simulink model "ResonantLLCConverter_continuous"  (R2024b)
settings: Solver=FixedStepAuto  StartTime=0.0  StopTime=tfinal  MaxStep=1e-4  RelTol=1e-6  EnableMultiTasking=on
PreLoadFcn:
  | Rs_fet=1e8;  % FET snubber resistance (ohms)
  | Cs_fet=inf;  % FET snubber capacitance (ohms)
  | Vf=0.6;        % Diode forward voltage (V)
libraries: spsDiodeLib x6, spsSeriesRLCBranchLib x3, spsCurrentMeasurementLib x3, spsIGBTDiodeLib x2, spsIdealSwitchLib x2, spsOnDelayLib x2, spsVoltageMeasurementLib x2, spsLinearTransformerLib x1, spsControlledVoltageSourceLib x1, sps_lib x1
settings Model: SimulationMode=accelerator  Creator=The MathWorks, Inc.  LastModifiedBy=XixiLab
settings SolverCC: AlgebraicLoopSolver=TrustRegion  SolverResetMethod=Robust  EnableFixedStepZeroCrossing=on
settings DataIOCC: SaveFormat=Array  SaveState=on  ReturnWorkspaceOutputs=off
settings OptimizationCC: LifeSpan=inf
settings DebuggingCC: ReadBeforeWriteMsg=DisableAll  WriteAfterWriteMsg=DisableAll  WriteAfterReadMsg=DisableAll  MultiTaskDSMMsg=none  UnconnectedInputMsg=warning  UnconnectedOutputMsg=warning  UnconnectedLineMsg=warning  SFUnexpectedBacktrackingDiag=warning  SFNoUnconditionalDefaultTransitionDiag=warning  SFExecutionAtInitializationDiag=none  ArithmeticOperatorsInVariantConditions=warning
settings ModelReferenceCC: UpdateModelReferenceTargets=IfOutOfDate  EnableRefExpFcnMdlSchedulingChecks=on
settings SFSimCC: SFSimEcho=off  SimUseLocalCustomCode=off  CustomCodeUndefinedFunction=UseInterfaceOnly
settings RTWCC: RTWUseLocalCustomCode=off  GPUComputeCapability=3.5
settings CodeAppCC: StateflowObjectComments=on
settings GRTTargetCC: TargetLangStandard=C89/C90 (ANSI)
settings ConfigComp: CovMetricSettings=dw  CovSaveCumulativeToWorkspaceVar=on  CovSaveSingleToWorkspaceVar=on  CovExternalEMLEnable=off
settings SimscapeCC: SimscapeNormalizeSystem=off  SimscapeNominalValues={1, 'bar'; 1, 'cm^3/s'; 1, 'bar*kg/s'; 1, 'kJ/kg'; 1, 'kW'; }

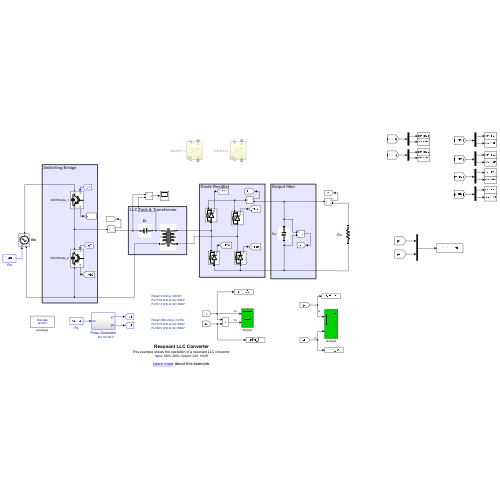
[thumbnail: Simulink's stored preview of the top-level diagram]
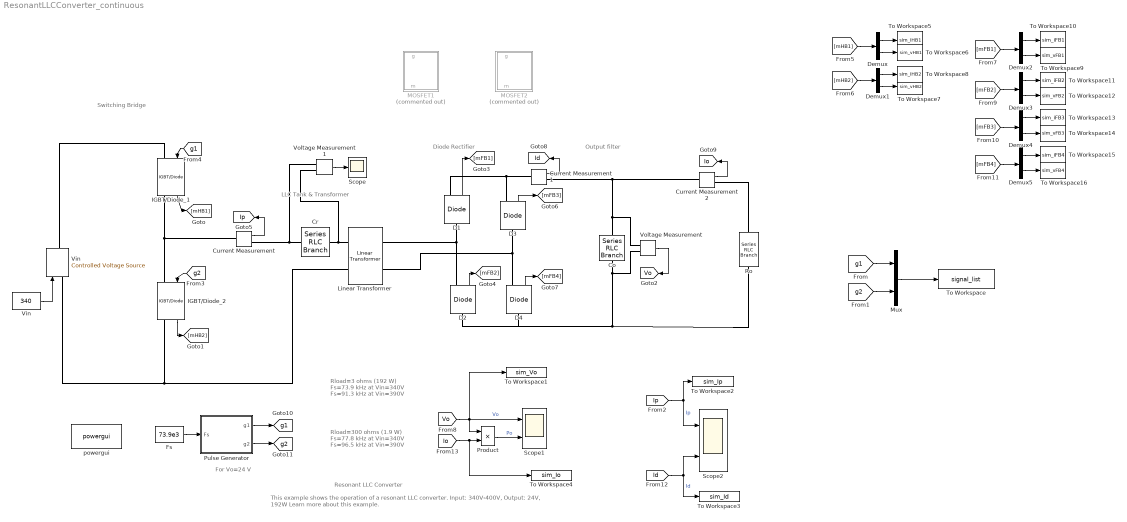
== system ResonantLLCConverter_continuous ==
  note: For Vo=24 V
  note: Rload=300 ohms (1.9 W)
      | Fs=77.8 kHz at Vin=340V
      | Fs=96.5 kHz at Vin=390V
  note: Diode Rectifier
  note: Switching Bridge
  note: Output filter
  note: LLC Tank & Transformer
  note: Rload=3 ohms (192 W)
      | Fs=73.9 kHz at Vin=340V
      | Fs=91.3 kHz at Vin=390V
  note: Resonant LLC Converter
  note: This example shows the operation of a resonant LLC converter.
      | Input: 340V-400V, Output: 24V, 192W
      |
      | Learn more about this example.
  Co : spsSeriesRLCBranchLib/Series RLC Branch  LConnTagsString=__new0  RConnTagsString=__new0  BranchType=C  Resistance=1e-4  Inductance=200e-6  SetiL0=off  InitialCurrent=0  Capacitance=100e-6  Setx0=on  InitialVoltage=24  Measurements=None
  Cr : spsSeriesRLCBranchLib/Series RLC Branch  LConnTagsString=__new0  RConnTagsString=__new0  BranchType=C  Resistance=1e-4  Inductance=200e-6  SetiL0=off  InitialCurrent=0  Capacitance=15e-9  Setx0=off  InitialVoltage=40  Measurements=None
  Current Measurement : spsCurrentMeasurementLib/Current Measurement  PhasorSimulation=off  OutputType=Complex  PSBequivalent=0
  Current Measurement1 : spsCurrentMeasurementLib/Current Measurement  PhasorSimulation=off  OutputType=Complex  PSBequivalent=0
  Current Measurement2 : spsCurrentMeasurementLib/Current Measurement  PhasorSimulation=off  OutputType=Complex  PSBequivalent=0
  D{1..4} (4 alike) : spsDiodeLib/Diode  Ron=1e-3  Lon=0  Vf=0.5  IC=0  UseSnubber=off  Rs=1e6  Cs=inf  Measurements=on
  Demux{,1..5} (6 alike) : Demux  Outputs=2
  Fs : Constant  Value=73.9e3
  IGBT/Diode_1 : spsIGBTDiodeLib/IGBT//Diode  Ron=1e-3  Rs=Rs_fet  Cs=Cs_fet  Measurements=on
  IGBT/Diode_2 : spsIGBTDiodeLib/IGBT//Diode  Ron=1e-3  Rs=Rs_fet  Cs=Cs_fet  Measurements=on
  Linear Transformer : spsLinearTransformerLib/Linear Transformer  UNITS=SI  NominalPower=[ 200 85e3 ]  winding1="[52   1e-2  102e-6]"  winding2="[6  1e-2  1.36e-6 ]"  ThreeWindings=off  winding3=[3.15e+05 0.7938 0.084225]  RmLm=[1e4 963e-6]  Measurements=None  DataType=on
  MOSFET1 : Subsystem  Commented=on
  MOSFET2 : Subsystem  Commented=on
  Mux : Mux  Inputs=2
  Product : Product
  Pulse Generator : Subsystem
  Ro : spsSeriesRLCBranchLib/Series RLC Branch  LConnTagsString=__new0  RConnTagsString=__new0  BranchType=R  Resistance=3  Inductance=200e-6  SetiL0=off  InitialCurrent=0  Capacitance=400e-6  Setx0=off  InitialVoltage=0  Measurements=None
  Scope : Scope
  Scope1 : Scope  NumInputPorts=2
  Scope2 : Scope  NumInputPorts=2
  To Workspace : ToWorkspace  VariableName=signal_list  SampleTime=-1
      settings: Save2DSignal=2-D array (concatenate along first dimension)
  To Workspace1 : ToWorkspace  VariableName=sim_Vo  SampleTime=-1
      settings: Save2DSignal=2-D array (concatenate along first dimension)
  To Workspace10 : ToWorkspace  VariableName=sim_iFB1  SampleTime=-1
      settings: Save2DSignal=2-D array (concatenate along first dimension)
  To Workspace11 : ToWorkspace  VariableName=sim_iFB2  SampleTime=-1
      settings: Save2DSignal=2-D array (concatenate along first dimension)
  To Workspace12 : ToWorkspace  VariableName=sim_vFB2  SampleTime=-1
      settings: Save2DSignal=2-D array (concatenate along first dimension)
  To Workspace13 : ToWorkspace  VariableName=sim_iFB3  SampleTime=-1
      settings: Save2DSignal=2-D array (concatenate along first dimension)
  To Workspace14 : ToWorkspace  VariableName=sim_vFB3  SampleTime=-1
      settings: Save2DSignal=2-D array (concatenate along first dimension)
  To Workspace15 : ToWorkspace  VariableName=sim_iFB4  SampleTime=-1
      settings: Save2DSignal=2-D array (concatenate along first dimension)
  To Workspace16 : ToWorkspace  VariableName=sim_vFB4  SampleTime=-1
      settings: Save2DSignal=2-D array (concatenate along first dimension)
  To Workspace2 : ToWorkspace  VariableName=sim_Ip  SampleTime=-1
      settings: Save2DSignal=2-D array (concatenate along first dimension)
  To Workspace3 : ToWorkspace  VariableName=sim_Id  SampleTime=-1
      settings: Save2DSignal=2-D array (concatenate along first dimension)
  To Workspace4 : ToWorkspace  VariableName=sim_Io  SampleTime=-1
      settings: Save2DSignal=2-D array (concatenate along first dimension)
  To Workspace5 : ToWorkspace  VariableName=sim_iHB1  SampleTime=-1
      settings: Save2DSignal=2-D array (concatenate along first dimension)
  To Workspace6 : ToWorkspace  VariableName=sim_vHB1  SampleTime=-1
      settings: Save2DSignal=2-D array (concatenate along first dimension)
  To Workspace7 : ToWorkspace  VariableName=sim_vHB2  SampleTime=-1
      settings: Save2DSignal=2-D array (concatenate along first dimension)
  To Workspace8 : ToWorkspace  VariableName=sim_iHB2  SampleTime=-1
      settings: Save2DSignal=2-D array (concatenate along first dimension)
  To Workspace9 : ToWorkspace  VariableName=sim_vFB1  SampleTime=-1
      settings: Save2DSignal=2-D array (concatenate along first dimension)
  Vin : Constant  Value=340
  "Vin " : spsControlledVoltageSourceLib/Controlled Voltage Source  Initialize=on  Source_Type=AC  Amplitude=0  Phase=0  Frequency=0  Measurements=None
  Voltage Measurement : spsVoltageMeasurementLib/Voltage Measurement  PhasorSimulation=off  OutputType=Complex  PSBequivalent=0
  Voltage Measurement1 : spsVoltageMeasurementLib/Voltage Measurement  PhasorSimulation=off  OutputType=Complex  PSBequivalent=0
  powergui : sps_lib/powergui  Priority=1  SimulationMode=Discrete  SampleTime=1e-9  frequency=60  Iterations=50  frequencyindice=0  Pbase=100e6  ErrMax=1e-4  UnitsV=kV  UnitsW=MW  buscounter=0  FunctionMessages=off  echomessages=off  EnableUseOfTLC=off  CurrentSourceSwitches=off  DisableSnubberDevices=off  DisableRonSwitches=off  DisableVfSwitches=off  DisplayEquations=off  AutomaticDiscreteSolvers=off  SolverType=Tustin/Backward Euler (TBE)  Interpol=off  ExternalGateDelay=off  methode=off  Ts=10  x0status=blocks  SPID=on  SwTol=0  HookPort=off  NonlinearTolerance=0  nMaxIteration=15  ContinueOnMaxIteration=off  RestoreLinks=warning  ResistiveCurrentMeasurement=off  Frange=[0:2:500]  Ylog=off  Xlog=on  ShowGrid=off  save=off  variable=ZData  structure=0  ZoomFFT=off  StartTime=0.0  cycles=1  DisplayStyle=1  fundamental=60  FreqAxis=off  MaxFrequency=1000  frequencyindicesteady=1  RmsSteady=1  display=off
  tag scope: Id=global, Io=global, Ip=global, Vo=global, g1=global, g2=global
  wires:
  Current Measurement/1 -> [Ip]
  Voltage Measurement/1 -> [Vo]
  Current Measurement1/1 -> [Id]
  Current Measurement2/1 -> [Io]
  [Io] -> To Workspace4/1, Product/2
  Pulse Generator/1(g1) -> [g1]
  Pulse Generator/2(g2) -> [g2]
  Fs/1 -> Pulse Generator/1(Fs)
  Product/1 -> Scope1/2  "Po"
  [Vo] -> To Workspace1/1, Product/1, Scope1/1  "Vo"
  Vin/1 -> "Vin "/1
  [Id] -> Scope2/2, To Workspace3/1  "Id"
  [Ip] -> Scope2/1, To Workspace2/1  "Ip"
  [g1] -> Mux/1
  [g2] -> Mux/2
  Mux/1 -> To Workspace/1
  [g1] -> IGBT/Diode_1/1
  IGBT/Diode_1/1 -> [mHB1]
  [g2] -> IGBT/Diode_2/1
  IGBT/Diode_2/1 -> [mHB2]
  D1/1 -> [mFB1]
  D4/1 -> [mFB4]
  [mHB1] -> Demux/1
  [mHB2] -> Demux1/1
  [mFB1] -> Demux2/1
  Demux/1 -> To Workspace5/1
  Demux/2 -> To Workspace6/1
  [mFB2] -> Demux3/1
  [mFB3] -> Demux4/1
  [mFB4] -> Demux5/1
  Demux1/1 -> To Workspace8/1
  Demux1/2 -> To Workspace7/1
  Demux2/1 -> To Workspace10/1
  Demux2/2 -> To Workspace9/1
  Demux3/1 -> To Workspace11/1
  Demux3/2 -> To Workspace12/1
  Demux4/2 -> To Workspace14/1
  Demux4/1 -> To Workspace13/1
  Demux5/2 -> To Workspace16/1
  Demux5/1 -> To Workspace15/1
  D2/1 -> [mFB2]
  D3/1 -> [mFB3]
  Voltage Measurement1/1 -> Scope/1
  connections:
  Co/RConn1 -- Voltage Measurement/LConn2 -- D4/LConn1 -- D2/LConn1 -- Ro/RConn1
  Linear Transformer/RConn1 -- D2/RConn1 -- D1/LConn1
  IGBT/Diode_1/RConn1 -- IGBT/Diode_2/LConn1 -- Current Measurement/LConn1
  Linear Transformer/LConn2 -- IGBT/Diode_2/RConn1 -- "Vin "/LConn1
  Cr/LConn1 -- Voltage Measurement1/LConn1 -- Current Measurement/RConn1
  Linear Transformer/LConn1 -- Voltage Measurement1/LConn2 -- Cr/RConn1
  D1/RConn1 -- D3/RConn1 -- Current Measurement1/LConn1
  Voltage Measurement/LConn1 -- Current Measurement2/LConn1 -- Current Measurement1/RConn1 -- Co/LConn1
  Current Measurement2/RConn1 -- Ro/LConn1
  IGBT/Diode_1/LConn1 -- "Vin "/RConn1
  D3/LConn1 -- D4/RConn1 -- Linear Transformer/RConn2

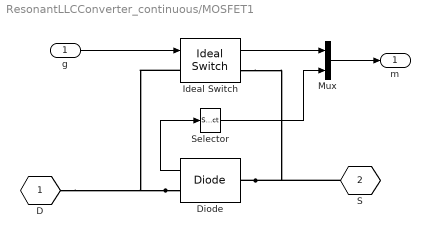
== system ResonantLLCConverter_continuous/MOSFET1 ==
  g : Inport
  Diode : spsDiodeLib/Diode  Ron=1e-3  Lon=0  Vf=0  IC=0  UseSnubber=0  Rs=inf  Cs=0  Measurements=on
  Ideal Switch : spsIdealSwitchLib/Ideal Switch  Ron=1e-3  Lon=0  IC=0  Rs=Rs_fet  Cs=Cs_fet  Measurements=on
  Mux : Mux  Inputs=[2,1]
  Selector : Selector  InputPortWidth=2  IndexOptions=Index vector (dialog)  Indices=1  OutputSizes=1
  D : PMIOPort  Tag=PMCPort  Side=Left
  S : PMIOPort  Tag=PMCPort  Port=2  Side=Right
  m : Outport  VectorParamsAs1DForOutWhenUnconnected=off
  wires:
  Diode/1 -> Selector/1
  g/1 -> Ideal Switch/1
  Ideal Switch/1 -> Mux/1
  Selector/1 -> Mux/2
  Mux/1 -> m/1
  connections:
  Diode/LConn1 -- S/RConn1 -- Ideal Switch/RConn1
  Diode/RConn1 -- D/RConn1 -- Ideal Switch/LConn1

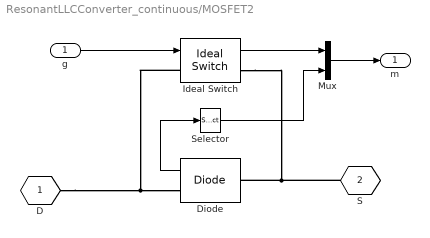
== system ResonantLLCConverter_continuous/MOSFET2 ==
  g : Inport
  Diode : spsDiodeLib/Diode  Ron=1e-3  Lon=0  Vf=0  IC=0  UseSnubber=0  Rs=inf  Cs=0  Measurements=on
  Ideal Switch : spsIdealSwitchLib/Ideal Switch  Ron=1e-3  Lon=0  IC=0  Rs=Rs_fet  Cs=Cs_fet  Measurements=on
  Mux : Mux  Inputs=[2,1]
  Selector : Selector  InputPortWidth=2  IndexOptions=Index vector (dialog)  Indices=1  OutputSizes=1
  D : PMIOPort  Tag=PMCPort  Side=Left
  S : PMIOPort  Tag=PMCPort  Port=2  Side=Right
  m : Outport  VectorParamsAs1DForOutWhenUnconnected=off
  wires:
  Mux/1 -> m/1
  Selector/1 -> Mux/2
  Ideal Switch/1 -> Mux/1
  g/1 -> Ideal Switch/1
  Diode/1 -> Selector/1
  connections:
  Ideal Switch/LConn1 -- D/RConn1 -- Diode/RConn1
  Ideal Switch/RConn1 -- S/RConn1 -- Diode/LConn1

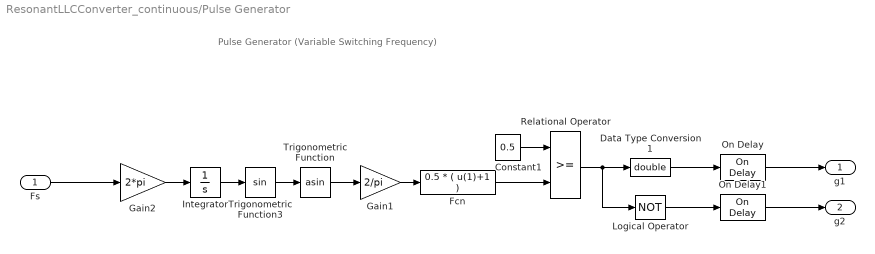
== system ResonantLLCConverter_continuous/Pulse Generator ==
  note: Pulse Generator
      | (Variable Switching Frequency)
  Fs : Inport
  Constant1 : Constant  Value=0.5
  Data Type Conversion1 : DataTypeConversion  OutDataTypeStr=double  SaturateOnIntegerOverflow=off  RndMeth=Floor
  Fcn : Fcn  Expr=0.5 * ( u(1)+1 )
  Gain1 : Gain  Gain=2/pi  SaturateOnIntegerOverflow=on  OutDataTypeStr=Inherit: Same as input  ParamDataTypeStr=Inherit: Same as input
  Gain2 : Gain  Gain=2*pi  SaturateOnIntegerOverflow=on  OutDataTypeStr=Inherit: Same as input  ParamDataTypeStr=Inherit: Same as input
  Integrator : Integrator
  Logical Operator : Logic  Operator=NOT  AllPortsSameDT=off  OutDataTypeStr=float('double')
  On Delay : spsOnDelayLib/On Delay  DelayType=On delay  delay=400e-9  ic=0  Ts=0
  On Delay1 : spsOnDelayLib/On Delay  DelayType=On delay  delay=400e-9  ic=0  Ts=0
  Relational Operator : RelationalOperator  OutDataTypeStr=boolean  InputSameDT=off
  Trigonometric Function : Trigonometry  Operator=asin
  Trigonometric Function3 : Trigonometry
  g1 : Outport  VectorParamsAs1DForOutWhenUnconnected=off
  g2 : Outport  Port=2  VectorParamsAs1DForOutWhenUnconnected=off
  wires:
  Trigonometric Function3/1 -> Trigonometric Function/1
  Gain1/1 -> Fcn/1
  Trigonometric Function/1 -> Gain1/1
  Integrator/1 -> Trigonometric Function3/1
  Constant1/1 -> Relational Operator/1
  Relational Operator/1 -> Data Type Conversion1/1, Logical Operator/1
  Fcn/1 -> Relational Operator/2
  Logical Operator/1 -> On Delay1/1
  Data Type Conversion1/1 -> On Delay/1
  Gain2/1 -> Integrator/1
  Fs/1 -> Gain2/1
  On Delay/1 -> g1/1
  On Delay1/1 -> g2/1
